simulink model "gesamtkonzept_p_regler"  (R2016b)
settings: Solver=ode1  StartTime=0.0  StopTime=Inf  FixedStep=0.001  RelTol=1e-3
PostLoadFcn:
  | , if any(exist('dsrtsu_mdlpostloadfcn', 'file') == [2, 3, 6]), try dsrtsu_mdlpostloadfcn('Execute', bdroot); catch fprintf('Error in PostLoadFcn (dsrtsu_mdlpostloadfcn) for model "%s":\n %s\n', bdroot, lasterr); end, end,
undefined symbols (not defined in the file): Continuous, matA_hub_g, matB_hub, matB_hub_g, matC_hub_g, matE_hub, matR_hub, reglerhub, Time
libraries: rti1202lib_adc_class1 x3, rti1202lib_dac_class1 x3, simulink_extras x1, ctrlSharedLib x1, simulink x1, rtiemclib x1, rti1202lib_base x1
(part 2 of 2)

== system gesamtkonzept_p_regler/Regler_Hub/Initial State ==
  In : Inport
  Trigger : TriggerPort  VariantControl=Variant
  Out : Outport
  wires:
  In/1 -> Out/1

== system gesamtkonzept_p_regler/Regler_Hub/kalman_on ==
  In : Inport
  Enable : EnablePort
  Out : Outport
  wires:
  In/1 -> Out/1

== system gesamtkonzept_p_regler/Regler_Hub/regler_on 3 ==
  regler_ on : Inport
  In : Inport  Port=2
  Signal Specification : SignalSpecification  Dimensions=1
  regler_on 2 : MATLABSystem  System=regler_switch_1  SimulateUsing=Code generation
      mask Type: regler_switch_1
      mask Display:
      | disp('regler_switch_1');
      | port_label('input',1,'regler_on');
      | port_label('input',2,'input');
      | port_label('output',1,'y');
  Out : Outport
  wires:
  regler_ on/1 -> regler_on 2/1
  regler_on 2/1 -> Out/1
  Signal Specification/1 -> regler_on 2/2
  In/1 -> Signal Specification/1

== system gesamtkonzept_p_regler/Regler_Hub/regler_on 4 ==
  regler_ on : Inport
  In : Inport  Port=2
  Signal Specification : SignalSpecification  Dimensions=1
  regler_on 2 : MATLABSystem  System=regler_switch_1  SimulateUsing=Code generation
      mask Type: regler_switch_1
      mask Display:
      | disp('regler_switch_1');
      | port_label('input',1,'regler_on');
      | port_label('input',2,'input');
      | port_label('output',1,'y');
  Out : Outport
  wires:
  regler_ on/1 -> regler_on 2/1
  regler_on 2/1 -> Out/1
  Signal Specification/1 -> regler_on 2/2
  In/1 -> Signal Specification/1

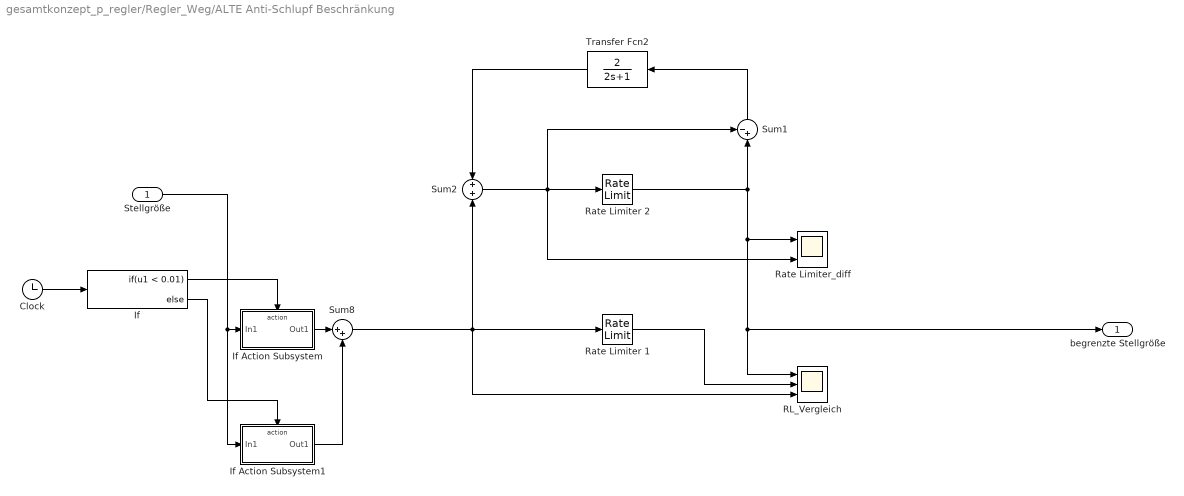
== system gesamtkonzept_p_regler/Regler_Weg/ALTE Anti-Schlupf Beschränkung ==
  Stellgröße : Inport
  Clock : Clock
  If : If  IfExpression=u1 < 0.01
  If Action Subsystem : Subsystem  TreatAsAtomicUnit=on
  If Action Subsystem1 : Subsystem  TreatAsAtomicUnit=on
  RL_Vergleich : Scope  NumInputPorts=3
  Rate Limiter 1 : RateLimiter  RisingSlewLimit=9.57  FallingSlewLimit=-9.57  SampleTimeMode=inherited
  Rate Limiter 2 : RateLimiter  RisingSlewLimit=9.57  FallingSlewLimit=-9.57  SampleTimeMode=inherited
  Rate Limiter_diff : Scope  NumInputPorts=2
  Sum1 : Sum  Inputs=-+|
  Sum2 : Sum  Inputs=+|+
  Sum8 : Sum  Inputs=|++
  Transfer Fcn2 : TransferFcn  Numerator=[2]  Denominator=[2 1]
  begrenzte Stellgröße : Outport
  wires:
  Stellgröße/1 -> If Action Subsystem1/1(In1), If Action Subsystem/1(In1)
  If Action Subsystem/1(Out1) -> Sum8/1
  If Action Subsystem1/1(Out1) -> Sum8/2
  Clock/1 -> If/1
  If/1 -> If Action Subsystem/Action
  If/2 -> If Action Subsystem1/Action
  Sum8/1 -> RL_Vergleich/3, Sum2/2, Rate Limiter 1/1
  Sum2/1 -> Rate Limiter_diff/2, Sum1/1, Rate Limiter 2/1
  Sum1/1 -> Transfer Fcn2/1
  Transfer Fcn2/1 -> Sum2/1
  Rate Limiter 2/1 -> begrenzte Stellgröße/1, RL_Vergleich/1, Rate Limiter_diff/1, Sum1/2
  Rate Limiter 1/1 -> RL_Vergleich/2

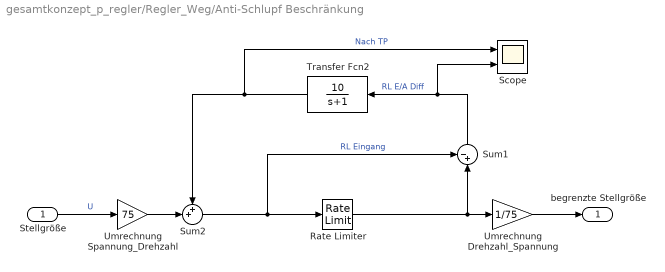
== system gesamtkonzept_p_regler/Regler_Weg/Anti-Schlupf Beschränkung ==
  Stellgröße : Inport
  Rate Limiter : RateLimiter  RisingSlewLimit=9.57  FallingSlewLimit=-9.57  SampleTimeMode=inherited
  Scope : Scope  NumInputPorts=2
  Sum1 : Sum  Inputs=-+|
  Sum2 : Sum  Inputs=++|
  Transfer Fcn2 : TransferFcn  Numerator=[10]  Denominator=[1 1]
  Umrechnung Drehzahl_Spannung : Gain  Gain=1/75
  Umrechnung Spannung_Drehzahl : Gain  Gain=75
  begrenzte Stellgröße : Outport
  wires:
  Stellgröße/1 -> Umrechnung Spannung_Drehzahl/1  "U"
  Sum2/1 -> Sum1/1, Rate Limiter/1  "RL Eingang"
  Sum1/1 -> Scope/2, Transfer Fcn2/1  "RL E/A Diff"
  Transfer Fcn2/1 -> Scope/1, Sum2/1  "Nach TP"
  Rate Limiter/1 -> Umrechnung Drehzahl_Spannung/1, Sum1/2
  Umrechnung Spannung_Drehzahl/1 -> Sum2/2
  Umrechnung Drehzahl_Spannung/1 -> begrenzte Stellgröße/1

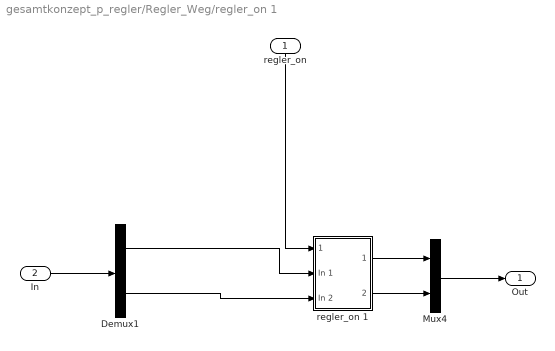
== system gesamtkonzept_p_regler/Regler_Weg/regler_on 1 ==
  regler_on : Inport
  In : Inport  Port=2
  Demux1 : Demux  Outputs=2
  Mux4 : Mux  Inputs=2
  regler_on 1 : Subsystem
  Out : Outport
  wires:
  Demux1/1 -> regler_on 1/2(In 1)
  Demux1/2 -> regler_on 1/3(In 2)
  regler_on 1/2(Out 2) -> Mux4/2
  regler_on 1/1(Out 1) -> Mux4/1
  Mux4/1 -> Out/1
  regler_on/1 -> regler_on 1/1(regler_ on)
  In/1 -> Demux1/1

== system gesamtkonzept_p_regler/Regler_Weg/regler_on 2 ==
  regler_ on : Inport
  In : Inport  Port=2
  Signal Specification : SignalSpecification  Dimensions=1
  regler_on 2 : MATLABSystem  System=regler_switch_1  SimulateUsing=Code generation
      mask Type: regler_switch_1
      mask Display:
      | disp('regler_switch_1');
      | port_label('input',1,'regler_on');
      | port_label('input',2,'input');
      | port_label('output',1,'y');
  Out : Outport
  wires:
  regler_ on/1 -> regler_on 2/1
  regler_on 2/1 -> Out/1
  Signal Specification/1 -> regler_on 2/2
  In/1 -> Signal Specification/1

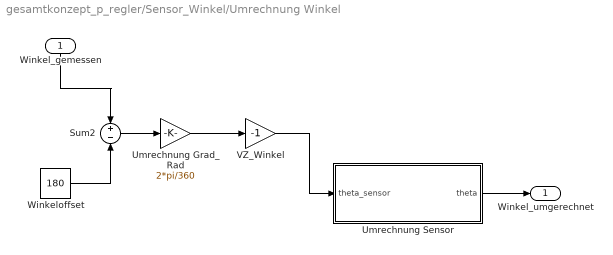
== system gesamtkonzept_p_regler/Sensor_Winkel/Umrechnung Winkel ==
  Winkel_gemessen : Inport
  Sum2 : Sum  Inputs=+|-
  Umrechnung Grad_Rad : Gain  Gain=2*pi/360
  Umrechnung Sensor : MATLAB Function  TreatAsAtomicUnit=on
  VZ_Winkel : Gain  Gain=-1
  Winkeloffset : Constant  Value=180
  Winkel_umgerechnet : Outport
  wires:
  Winkel_gemessen/1 -> Sum2/1
  VZ_Winkel/1 -> Umrechnung Sensor/1(theta_sensor)
  Winkeloffset/1 -> Sum2/2
  Sum2/1 -> Umrechnung Grad_Rad/1
  Umrechnung Grad_Rad/1 -> VZ_Winkel/1
  Umrechnung Sensor/1(theta) -> Winkel_umgerechnet/1

== system gesamtkonzept_p_regler/RTI Data/RTI Data Store/RTI Data Store ==
  RTI Data Store : Subsystem  mask(RTI_DATA_STORE){}
      mask help:
      | RTI Data Store Block. This block is used by RTI to store internal model dependent data. Deleting this block will result in data loss.
      |
      | NEVER DELETE, COPY, OR MODIFY THIS BLOCK!
      mask Help:
      | RTI Data Store Block. This block is used by RTI to store internal model dependent data. Deleting this block will result in data loss.
      | 
      | NEVER DELETE, COPY, OR MODIFY THIS BLOCK!
      mask Display: text(0.5, 0.5, ' ', 'HorizontalAlignment', 'center');

== system gesamtkonzept_p_regler/Regler_Weg/ALTE Anti-Schlupf Beschränkung/If Action Subsystem ==
  In1 : Inport
  Action Port : ActionPort
  Gain : Gain  Gain=0
  Out1 : Outport
  wires:
  In1/1 -> Gain/1
  Gain/1 -> Out1/1

== system gesamtkonzept_p_regler/Regler_Weg/ALTE Anti-Schlupf Beschränkung/If Action Subsystem1 ==
  In1 : Inport
  Action Port : ActionPort
  Gain : Gain
  Out1 : Outport
  wires:
  In1/1 -> Gain/1
  Gain/1 -> Out1/1

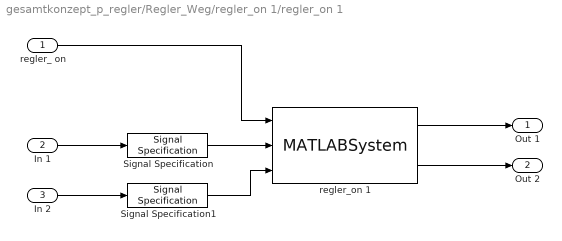
== system gesamtkonzept_p_regler/Regler_Weg/regler_on 1/regler_on 1 ==
  regler_ on : Inport
  In 1 : Inport  Port=2
  In 2 : Inport  Port=3
  Signal Specification : SignalSpecification  Dimensions=1
  Signal Specification1 : SignalSpecification  Dimensions=1
  regler_on 1 : MATLABSystem  System=regler_switch_2  SimulateUsing=Code generation
      mask Type: regler_switch_2
      mask Display:
      | disp('regler_switch_2');
      | port_label('input',1,'regler_on');
      | port_label('input',2,'input1');
      | port_label('input',3,'input2');
      | port_label('output',1,'y1');
      | port_label('output',2,'y2');
  Out 1 : Outport
  Out 2 : Outport  Port=2
  wires:
  regler_on 1/1 -> Out 1/1
  regler_on 1/2 -> Out 2/1
  In 2/1 -> Signal Specification1/1
  In 1/1 -> Signal Specification/1
  Signal Specification/1 -> regler_on 1/2
  Signal Specification1/1 -> regler_on 1/3
  regler_ on/1 -> regler_on 1/1

== system gesamtkonzept_p_regler/RTI Data/RTI Data Store/RTI Data Store/RTI Data Store ==
  RTI Data Store : Subsystem  mask(RTI_DATA_STORE){}
      mask help:
      | RTI Data Store Block. This block is used by RTI to store internal model dependent data. Deleting this block will result in data loss.
      |
      | NEVER DELETE, COPY, OR MODIFY THIS BLOCK!
      mask Help:
      | RTI Data Store Block. This block is used by RTI to store internal model dependent data. Deleting this block will result in data loss.
      | 
      | NEVER DELETE, COPY, OR MODIFY THIS BLOCK!
      mask Display: text(0.5, 0.5, ' ', 'HorizontalAlignment', 'center');

== system gesamtkonzept_p_regler/RTI Data/RTI Data Store/RTI Data Store/RTI Data Store/RTI Data Store ==

== matlab function gesamtkonzept_p_regler/Sensor_Winkel/Umrechnung Winkel/Umrechnung Sensor ==
  data: theta_sensor input; theta output
function theta  = sensorWinkel(theta_sensor)
% berechnet aus dem gemessenen Winkel den tatsächlichen Winkel des
% Lasthebers

% l_verb: Länge des Verbindungsstücks
% l_welle: Abstand der beiden Wellen

% Parameter für die Winkelumrechnung
l_verb = 0.109; % m %
l_welle = 0.0575; % m %

theta = asin(sin(theta_sensor) * (l_verb / sqrt(l_welle^2 + l_verb^2 - (2 * l_verb * l_welle * cos(theta_sensor)))));
